simulink model "TrafficLightController_SIL_Test"  (R2024b)
settings: Solver=VariableStepAuto  StartTime=0.0  StopTime=10.0  RelTol=1e-3
libraries: SignalEditorBlockLib x1
settings Model: Creator=adetunji  LastModifiedBy=adetunji

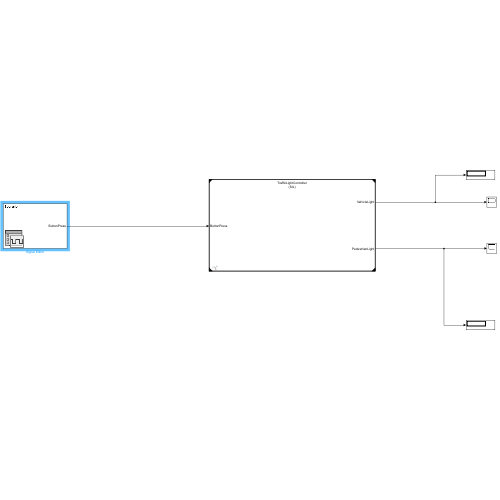
[thumbnail: Simulink's stored preview of the top-level diagram]
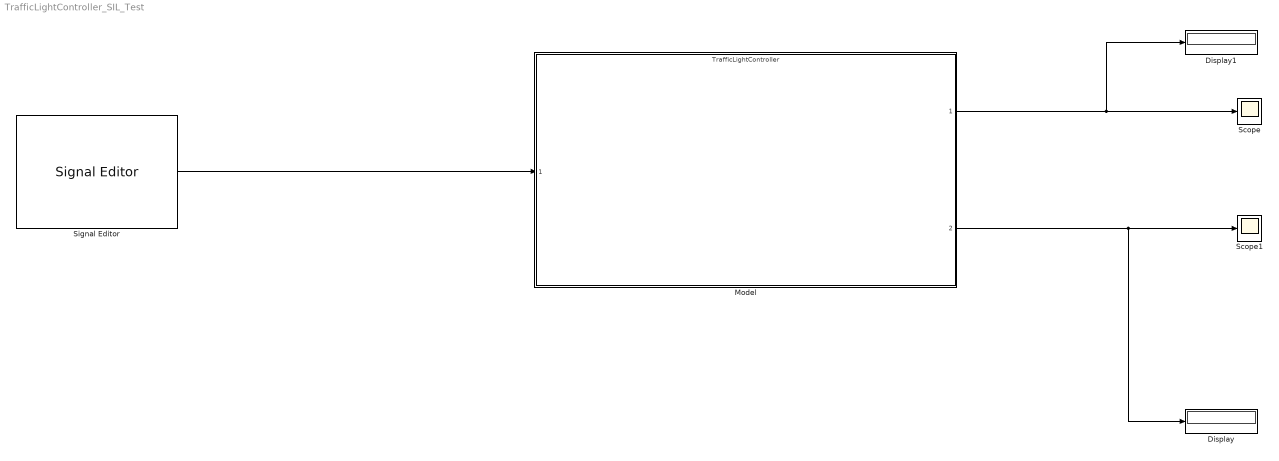
== system TrafficLightController_SIL_Test ==
  Display : Display
  Display1 : Display
  Model : ModelReference  ModelNameDialog=TrafficLightController  SimulationMode=Software-in-the-loop (SIL)  ModelReferenceVersion=1.1
  Scope : Scope
  Scope1 : Scope
  Signal Editor : SignalEditorBlockLib/Signal Editor  FileName=ButtonPress.mat  ActiveScenario=Scenario  ActiveSignal=ButtonPress  IsBus=off  OutputBusObjectStr=Bus: BusObject  SampleTime=0  Interpolate=off  ZeroCross=off  OutputAfterFinalValue=Setting to zero  Unit=inherit  PreserveSignalName=on  ApplySigPropsToAllScenarios=on  ApplySigPropsToAllSignals=off
  wires:
  Signal Editor/1 -> Model/1
  Model/2 -> Display/1, Scope1/1
  Model/1 -> Display1/1, Scope/1
